simulink model "line_sim_withoutConstraint"  (R2021b)
settings: Solver=ode4  StartTime=0.0  StopTime=10.0  FixedStep=0.01  RelTol=1e-3
undefined symbols (not defined in the file or in its folder): q0, q0dot
settings Model: Creator=Ramin_hp  LastModifiedBy=Rita
settings SolverCC: AlgebraicLoopSolver=TrustRegion
settings DataIOCC: ReturnWorkspaceOutputs=off
settings DebuggingCC: SFMachineParentedDataDiag=warning  ArithmeticOperatorsInVariantConditions=warning
settings SFSimCC: SimUseLocalCustomCode=off  CustomCodeUndefinedFunction=UseInterfaceOnly
settings RTWCC: RTWUseLocalCustomCode=off
settings CodeAppCC: StateflowObjectComments=on

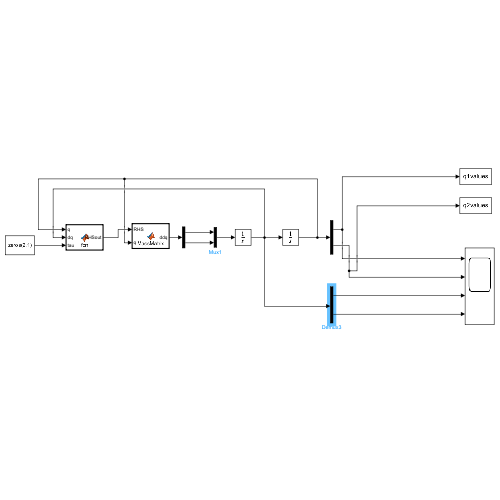
[thumbnail: Simulink's stored preview of the top-level diagram]
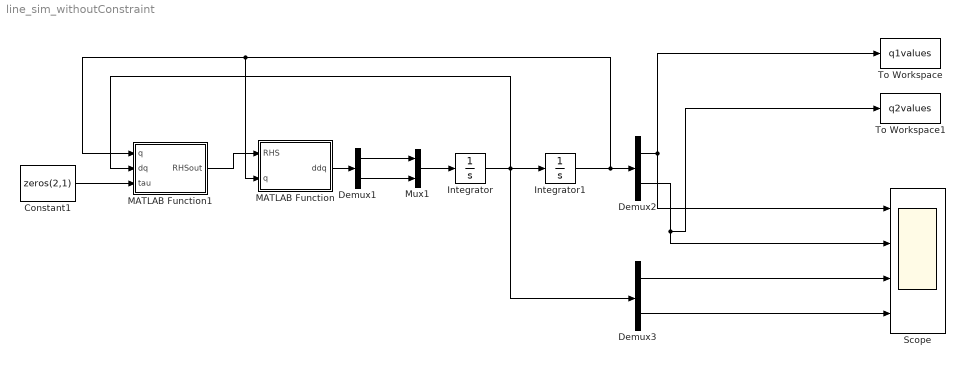
== system line_sim_withoutConstraint ==
  Constant1 : Constant  Value=zeros(2,1)
  Demux1 : Demux  Outputs=2
  Demux2 : Demux  Outputs=2
  Demux3 : Demux  Outputs=2
  Integrator : Integrator  InitialCondition=q0dot
  Integrator1 : Integrator  InitialCondition=q0
  MATLAB Function : MATLAB Function  TreatAsAtomicUnit=on
  MATLAB Function1 : MATLAB Function  TreatAsAtomicUnit=on
  Mux1 : Mux  Inputs=2
  Scope : Scope  NumInputPorts=4
  To Workspace : ToWorkspace  VariableName=q1values  SaveFormat=Timeseries  SampleTime=-1
  To Workspace1 : ToWorkspace  VariableName=q2values  SaveFormat=Timeseries  SampleTime=-1
  wires:
  Integrator/1 -> Demux3/1, Integrator1/1, MATLAB Function1/2(dq)
  Integrator1/1 -> MATLAB Function1/1(q), MATLAB Function/2(q), Demux2/1
  Demux2/1 -> To Workspace/1, Scope/1
  Demux2/2 -> To Workspace1/1, Scope/2
  Demux3/1 -> Scope/3
  Demux3/2 -> Scope/4
  MATLAB Function/1(ddq) -> Demux1/1
  Demux1/1 -> Mux1/1
  Demux1/2 -> Mux1/2
  Mux1/1 -> Integrator/1
  MATLAB Function1/1(RHSout) -> MATLAB Function/1(RHS)
  Constant1/1 -> MATLAB Function1/3(tau)

== matlab function line_sim_withoutConstraint/MATLAB Function ==
  data: RHS input; q input; ddq output
function ddq = MassMatrix(RHS,q)

IM = inertiaMatrix(q);

ddq = IM\RHS;

== matlab function line_sim_withoutConstraint/MATLAB Function1 ==
  data: q input; RHSout output; dq input; tau input
function RHSout = fcn(q,dq,tau)

RHSout = RHS_withoutConstraint(q,dq,tau);
